simulink model "AcDc"  (R2020b)
settings: Solver=FixedStepAuto  StartTime=0.0  StopTime=0.1  FixedStep=10e-5  RelTol=1e-3
libraries: powerlib x20, dspstat3 x5, powerlib_meascontrol x1
settings Model: Creator=New-life  LastModifiedBy=New-life

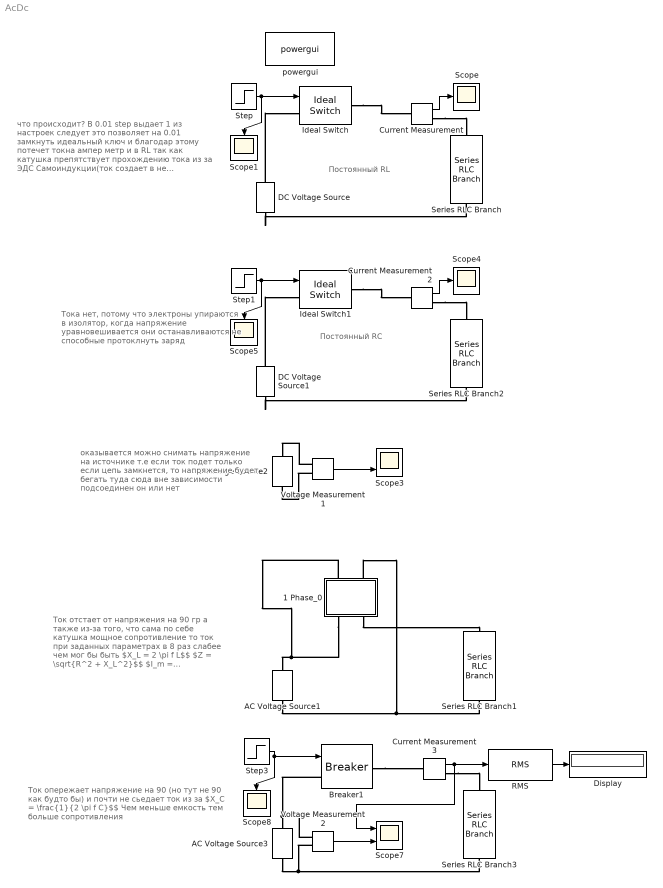
== system AcDc ==
  note: Ток опережает напряжение на 90
      | (но тут не 90 как будто бы) и почти не сьедает
      | ток из за $X_C = \frac{1}{2 \pi f C}$$ Чем меньше емкость тем
      | больше сопротивления
  note: Ток отстает от напряжения на 90 гр
      | а также из-за того, что сама по себе
      | катушка мощное сопротивление
      | то ток при заданных параметрах в
      | 8 раз слабее чем мог бы быть
      | $X_L = 2 \pi f L$$ $Z = \sqrt{R^2 + X_L^2}$$ $I_m = \frac{U_m}{Z}$$
      | ток в катушке стартовал с 0
      | а потом он устанавливается
  note: Постоянный RC
  note: Тока нет, потому что электроны
      | упираются в изолятор, когда напряжение
      | уравновешивается они останавливаются
      | не способные протоклнуть заряд
  note: оказывается можно снимать
      | напряжение на источнике
      | т.е если ток подет только если
      | цепь замкнется, то напряжение
      | будет бегать туда сюда вне зависимости
      | подсоединен он или нет
  note: что происходит? В 0.01 step выдает 1 из
      | настроек следует это позволяет на 0.01
      | замкнуть идеальный ключ и благодар
      | этому потечет токна ампер метр и в RL
      | так как катушка препятствует прохождению
      | тока из за ЭДС Самоиндукции(ток создает
      | в не элеткромагнитное поле), и течение тока
      | замедляется, он нарастает не мгновенно
  note: Постоянный RL
  1 Phase_0 : Subsystem
      settings: CopyFcn=|
      | % Получаем путь и имя нового (только что скопированного) блока
      | blockPath = gcb;
      | blockName = get_param(blockPath, 'Name');
      | 
      | % Ищем число в названии самой подсистемы (например, берем "2" из "Measure_2")
      | numStr = regexp(blockName, '\d+', 'match');
      | 
      | if ~isempty(numStr)
      |     newNum = numStr{end}; % Берем последнее найденное число
      | 
      |     % --- 1. Обновляем скрытые теги в Goto и From (радиочастоты) ---
      |     gotos = find_system(blockPath, 'LookUnderMasks', 'on', 'BlockType', 'Goto');
      |     froms = find_system(blockPath, 'LookUnderMasks', 'on', 'BlockType', 'From');
      | 
      |     for i = 1:length(gotos)
      |         oldTag = get_param(gotos{i}, 'GotoTag');
      |         set_param(gotos{i}, 'GotoTag', regexprep(oldTag, '\d+$', newNum));
      |     end
      |     for i = 1:length(froms)
      |         oldTag = get_param(froms{i}, 'GotoTag');
      |         set_param(froms{i}, 'GotoTag', regexprep(oldTag, '\d+$', newNum));
      |     end
      | 
      |     % --- 2. ПЕРЕИМЕНОВЫВАЕМ САМИ БЛОКИ (визуальные надписи UI0 -> UI1 и т.д.) ---
      |     % Ищем все элементы только внутри этой подсистемы
      |     internalBlocks = find_system(blockPath, 'SearchDepth', 1, 'LookUnderMasks', 'on');
      | 
      |     % Цикл начинаем с 2, так как 1-й элемент в списке - это сама папка подсистемы
      |     for i = 2:length(internalBlocks)
      |         oldName = get_param(internalBlocks{i}, 'Name');
      |         % Ищем цифру в конце имени и меняем на новую
      |         newName = regexprep(oldName, '\d+$', newNum);
      | 
      |         % Если имя изменилось, применяем его
      |         if ~strcmp(oldName, newName)
      |             try
      |                 set_param(internalBlocks{i}, 'Name', newName);
      |             catch
      |                 % Игнорируем ошибку, если вдруг такое имя уже случайно есть
      |             end
      |         end
      |     end
      | end
  AC Voltage Source1 : powerlib/Electrical Sources/AC Voltage Source  Amplitude=100  Phase=0  Frequency=50  SampleTime=0  Measurements=None  BusType=swing  Pref=10e3  Qref=0  Qmin=-inf  Qmax=+inf
  AC Voltage Source2 : powerlib/Electrical Sources/AC Voltage Source  Amplitude=100  Phase=0  Frequency=50  SampleTime=0  Measurements=None  BusType=swing  Pref=10e3  Qref=0  Qmin=-inf  Qmax=+inf
  AC Voltage Source3 : powerlib/Electrical Sources/AC Voltage Source  Amplitude=100  Phase=0  Frequency=50  SampleTime=0  Measurements=None  BusType=swing  Pref=10e3  Qref=0  Qmin=-inf  Qmax=+inf
  Breaker1 : powerlib/Elements/Breaker  InitialState=0  SwitchingTimes="[1/60  5/60]"  External=on  BreakerResistance=0.01  SnubberResistance=1e6  SnubberCapacitance=inf  Measurements=None  MoreParameters=on  NoBreakLoop=off
  Current Measurement : powerlib/Measurements/Current Measurement  PhasorSimulation=off  OutputType=Complex  PSBequivalent=0
  Current Measurement2 : powerlib/Measurements/Current Measurement  PhasorSimulation=off  OutputType=Complex  PSBequivalent=0
  Current Measurement3 : powerlib/Measurements/Current Measurement  PhasorSimulation=off  OutputType=Complex  PSBequivalent=0
  DC Voltage Source : powerlib/Electrical Sources/DC Voltage Source  Amplitude=100  Measurements=None
  DC Voltage Source1 : powerlib/Electrical Sources/DC Voltage Source  Amplitude=100  Measurements=None
  Display : Display
  Ideal Switch : powerlib/Power Electronics/Ideal Switch  Ron=0.01  Lon=0  IC=0  Rs=1e6  Cs=inf  Measurements=off
  Ideal Switch1 : powerlib/Power Electronics/Ideal Switch  Ron=0.01  Lon=0  IC=0  Rs=1e6  Cs=inf  Measurements=off
  RMS : dspstat3/RMS  run=off  directionMode=Each column  dimension=1  InputProcessing=Columns as channels (frame based)  reset_popup=None
  Scope{,1,4..5,8} (5 alike) : Scope
  Scope3 : Scope  NumInputPorts=2
  Scope7 : Scope  NumInputPorts=2
  Series RLC Branch : powerlib/Elements/Series RLC Branch  LConnTagsString=__new0  RConnTagsString=__new0  BranchType=RL  Resistance=0.5  Inductance=10e-3  SetiL0=off  InitialCurrent=0  Capacitance=1e-2  Setx0=off  InitialVoltage=0  Measurements=None
  Series RLC Branch1 : powerlib/Elements/Series RLC Branch  LConnTagsString=__new0  RConnTagsString=__new0  BranchType=RL  Resistance=0.5  Inductance=10e-3  SetiL0=on  InitialCurrent=0  Capacitance=10e-3  Setx0=off  InitialVoltage=0  Measurements=None
  Series RLC Branch2 : powerlib/Elements/Series RLC Branch  LConnTagsString=__new0  RConnTagsString=__new0  BranchType=RC  Resistance=0.5  Inductance=10e-3  SetiL0=off  InitialCurrent=0  Capacitance=1e-2  Setx0=off  InitialVoltage=0  Measurements=None
  Series RLC Branch3 : powerlib/Elements/Series RLC Branch  LConnTagsString=__new0  RConnTagsString=__new0  BranchType=RC  Resistance=0.5  Inductance=10e-3  SetiL0=on  InitialCurrent=0  Capacitance=10e-4  Setx0=off  InitialVoltage=0  Measurements=None
  Step : Step  Time=0.01  SampleTime=0
  Step1 : Step  Time=0.01  SampleTime=0
  Step3 : Step  Time=0.03  SampleTime=0
  Voltage Measurement1 : powerlib/Measurements/Voltage Measurement  PhasorSimulation=off  OutputType=Complex  PSBequivalent=0
  Voltage Measurement2 : powerlib/Measurements/Voltage Measurement  PhasorSimulation=off  OutputType=Complex  PSBequivalent=0
  powergui : powerlib/powergui  Priority=1  SimulationMode=Continuous  SampleTime=50e-6  frequency=60  Iterations=50  frequencyindice=50  Pbase=100e6  ErrMax=1e-4  UnitsV=kV  UnitsW=MW  buscounter=0  FunctionMessages=off  echomessages=off  EnableUseOfTLC=off  CurrentSourceSwitches=off  DisableSnubberDevices=off  DisableRonSwitches=off  DisableVfSwitches=off  DisplayEquations=off  AutomaticDiscreteSolvers=off  SolverType=Tustin/Backward Euler (TBE)  Interpol=off  ExternalGateDelay=off  methode=off  Ts=100  x0status=blocks  SPID=on  SwTol=0  HookPort=off  NonlinearTolerance=1e-4  nMaxIteration=100  ContinueOnMaxIteration=off  RestoreLinks=warning  ResistiveCurrentMeasurement=off  Frange=[0:2:500]  Ylog=off  Xlog=on  ShowGrid=off  save=off  variable=ZData  structure=0  ZoomFFT=off  StartTime=0.0  cycles=1  DisplayStyle=1  fundamental=60  FreqAxis=off  MaxFrequency=1000  frequencyindicesteady=1  RmsSteady=1  display=off
  wires:
  Current Measurement/1 -> Scope/1
  Step/1 -> Scope1/1, Ideal Switch/1
  Voltage Measurement1/1 -> Scope3/2
  Step1/1 -> Ideal Switch1/1, Scope5/1
  Current Measurement2/1 -> Scope4/1
  Step3/1 -> Scope8/1, Breaker1/1
  Voltage Measurement2/1 -> Scope7/2
  Current Measurement3/1 -> RMS/1, Scope7/1
  RMS/1 -> Display/1
  connections:
  1 Phase_0/RConn2 -- Series RLC Branch1/LConn1
  AC Voltage Source1/LConn1 -- 1 Phase_0/LConn2 -- Series RLC Branch1/RConn1
  Current Measurement/RConn1 -- Series RLC Branch/LConn1
  DC Voltage Source/LConn1 -- Series RLC Branch/RConn1
  DC Voltage Source/RConn1 -- Ideal Switch/LConn1
  Ideal Switch/RConn1 -- Current Measurement/LConn1
  Voltage Measurement1/LConn2 -- AC Voltage Source2/LConn1
  Voltage Measurement1/LConn1 -- AC Voltage Source2/RConn1
  Ideal Switch1/RConn1 -- Current Measurement2/LConn1
  DC Voltage Source1/RConn1 -- Ideal Switch1/LConn1
  DC Voltage Source1/LConn1 -- Series RLC Branch2/RConn1
  Current Measurement2/RConn1 -- Series RLC Branch2/LConn1
  Voltage Measurement2/LConn2 -- AC Voltage Source3/LConn1 -- Series RLC Branch3/RConn1
  Breaker1/LConn1 -- AC Voltage Source3/RConn1 -- Voltage Measurement2/LConn1
  Current Measurement3/RConn1 -- Series RLC Branch3/LConn1
  Breaker1/RConn1 -- Current Measurement3/LConn1
  1 Phase_0/RConn1 -- 1 Phase_0/LConn1 -- AC Voltage Source1/RConn1

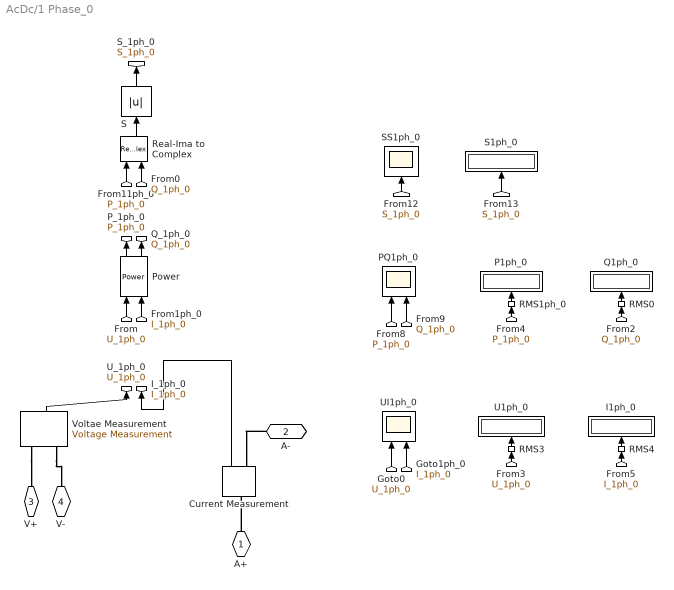
== system AcDc/1 Phase_0 ==
  Current Measurement : powerlib/Measurements/Current Measurement  PhasorSimulation=off  OutputType=Complex  PSBequivalent=0
  I1ph_0 : Display
      settings: Format=bank
  P1ph_0 : Display
      settings: Format=bank
  PQ1ph_0 : Scope  NumInputPorts=2
  Power : powerlib_meascontrol/Measurements/Power  Freq=60  Vinit=[1, 0]  Iinit=[1, 0]  Ts=0
  Q1ph_0 : Display
      settings: Format=bank
  RMS0 : dspstat3/RMS  run=off  directionMode=Each column  dimension=1  InputProcessing=Columns as channels (frame based)  reset_popup=None
  RMS1ph_0 : dspstat3/RMS  run=off  directionMode=Each column  dimension=1  InputProcessing=Columns as channels (frame based)  reset_popup=None
  RMS3 : dspstat3/RMS  run=off  directionMode=Each column  dimension=1  InputProcessing=Columns as channels (frame based)  reset_popup=None
  RMS4 : dspstat3/RMS  run=off  directionMode=Each column  dimension=1  InputProcessing=Columns as channels (frame based)  reset_popup=None
  Real-Ima to Complex : RealImagToComplex
  S : Abs
  S1ph_0 : Display
      settings: Format=bank
  SS1ph_0 : Scope
  U1ph_0 : Display
      settings: Format=bank
  UI1ph_0 : Scope  NumInputPorts=2
  Voltae Measurement : powerlib/Measurements/Voltage Measurement  PhasorSimulation=off  OutputType=Complex  PSBequivalent=0
  A+ : PMIOPort  Side=Right
  A- : PMIOPort  Port=2  Side=Right
  V+ : PMIOPort  Port=3  Side=Left
  V- : PMIOPort  Port=4  Side=Left
  tag scope: I_1ph_0=global, P_1ph_0=global, Q_1ph_0=global, S_1ph_0=global, U_1ph_0=global
  wires:
  Current Measurement/1 -> [I_1ph_0]
  Power/1 -> [P_1ph_0]
  Power/2 -> [Q_1ph_0]
  [I_1ph_0] -> Power/2
  [U_1ph_0] -> Power/1
  [Q_1ph_0] -> Real-Ima to Complex/2
  Voltae Measurement/1 -> [U_1ph_0]
  [I_1ph_0] -> UI1ph_0/2
  RMS4/1 -> I1ph_0/1
  [I_1ph_0] -> RMS4/1
  [Q_1ph_0] -> RMS0/1
  [P_1ph_0] -> Real-Ima to Complex/1
  RMS3/1 -> U1ph_0/1
  [U_1ph_0] -> RMS3/1
  RMS0/1 -> Q1ph_0/1
  RMS1ph_0/1 -> P1ph_0/1
  [P_1ph_0] -> RMS1ph_0/1
  [S_1ph_0] -> SS1ph_0/1
  [S_1ph_0] -> S1ph_0/1
  Real-Ima to Complex/1 -> S/1
  S/1 -> [S_1ph_0]
  [U_1ph_0] -> UI1ph_0/1
  [Q_1ph_0] -> PQ1ph_0/2
  [P_1ph_0] -> PQ1ph_0/1
  connections:
  A+/RConn1 -- Current Measurement/LConn1
  A-/RConn1 -- Current Measurement/RConn1
  Voltae Measurement/LConn2 -- V-/RConn1
  Voltae Measurement/LConn1 -- V+/RConn1
